simulink model "Computer"  (R2023a)
(part 2 of 6)

  Data_RAM (0x000 .. 0xFFF)/6(b6) -> Word_Enable35/7(b02)
  Data_RAM (0x000 .. 0xFFF)/1(b1) -> Word_Enable35/2(b07)
  Data_RAM (0x000 .. 0xFFF)/8(b8) -> Word_Enable35/9(b00)
  Data_RAM (0x000 .. 0xFFF)/3(b3) -> Word_Enable35/4(b05)
  Data_RAM (0x000 .. 0xFFF)/2(b2) -> Word_Enable35/3(b06)
  Data_ROM (0x000 .. 0xFFF)/2(b2) -> Word_Enable30/3(b06)
  Data_ROM (0x000 .. 0xFFF)/7(b7) -> Word_Enable30/8(b01)
  Data_ROM (0x000 .. 0xFFF)/6(b6) -> Word_Enable30/7(b02)
  Data_ROM (0x000 .. 0xFFF)/4(b4) -> Word_Enable30/5(b04)
  Data_ROM (0x000 .. 0xFFF)/1(b1) -> Word_Enable30/2(b07)
  Data_ROM (0x000 .. 0xFFF)/5(b5) -> Word_Enable30/6(b03)
  Data_ROM (0x000 .. 0xFFF)/3(b3) -> Word_Enable30/4(b05)
  Data_ROM (0x000 .. 0xFFF)/8(b8) -> Word_Enable30/9(b00)
  Word_Enable35/1("b07 ") -> Delay_8b/1
  Word_Enable35/2("b06 ") -> Delay_8b/2
  Word_Enable35/3("b05 ") -> Delay_8b/3
  Word_Enable35/4("b04 ") -> Delay_8b/4
  Word_Enable35/5("b03 ") -> Delay_8b/5
  Word_Enable35/6("b02 ") -> Delay_8b/6
  Word_Enable35/7("b01 ") -> Delay_8b/7
  Word_Enable35/8("b00 ") -> Delay_8b/8
  Merge2_8b_Simulated1/1 -> Merge2_8b_Simulated2/9
  Merge2_8b_Simulated1/2 -> Merge2_8b_Simulated2/10
  Merge2_8b_Simulated1/3 -> Merge2_8b_Simulated2/11
  Merge2_8b_Simulated1/4 -> Merge2_8b_Simulated2/12
  Merge2_8b_Simulated1/5 -> Merge2_8b_Simulated2/13
  Merge2_8b_Simulated1/6 -> Merge2_8b_Simulated2/14
  Merge2_8b_Simulated1/7 -> Merge2_8b_Simulated2/15
  Merge2_8b_Simulated1/8 -> Merge2_8b_Simulated2/16
  Align28/4 -> Video_RAM (0x000 .. 0x3FF)/69(Data_b04)
  Align28/3 -> Video_RAM (0x000 .. 0x3FF)/68(Data_b05)
  Align28/7 -> Video_RAM (0x000 .. 0x3FF)/72(Data_b01)
  Align28/6 -> Video_RAM (0x000 .. 0x3FF)/71(Data_b02)
  Align28/1 -> Video_RAM (0x000 .. 0x3FF)/66(Data_b07)
  Align28/2 -> Video_RAM (0x000 .. 0x3FF)/67(Data_b06)
  Align28/8 -> Video_RAM (0x000 .. 0x3FF)/73(Data_b00)
  Align28/5 -> Video_RAM (0x000 .. 0x3FF)/70(Data_b03)
  Align29/8 -> Align28/8
  Align29/7 -> Align28/7
  Align29/6 -> Align28/6
  Align29/5 -> Align28/5
  Align29/4 -> Align28/4
  Align29/3 -> Align28/3
  Align29/2 -> Align28/2
  Align29/1 -> Align28/1
  <0x2000..0x23FF>/1(Sel(1b)) -> Logical Operator26/2, Word_Enable27/1(Sel(1b))
  Align31/1 -> <0x2000..0x23FF>/1(b15)
  Align31/2 -> <0x2000..0x23FF>/2(b14)
  Align31/3 -> <0x2000..0x23FF>/3(b13)
  Align31/4 -> <0x2000..0x23FF>/4(b12)
  Align31/5 -> <0x2000..0x23FF>/5(b11)
  Align31/6 -> <0x2000..0x23FF>/6(b10), Dec_32_Enbl14/2
  Align31/7 -> Dec_32_Enbl14/3, <0x2000..0x23FF>/7(b09)
  Align31/8 -> <0x2000..0x23FF>/8(b08), Dec_32_Enbl14/4
  Align31/9 -> <0x2000..0x23FF>/9(b07), Dec_32_Enbl14/5
  Align31/10 -> Dec_32_Enbl14/6, <0x2000..0x23FF>/10(b06)
  Align31/11 -> <0x2000..0x23FF>/11(b05)
  Align31/12 -> <0x2000..0x23FF>/12(b04), Align32/5
  Align31/13 -> <0x2000..0x23FF>/13(b03), Align32/4
  Align31/14 -> <0x2000..0x23FF>/14(b02), Align32/3
  Align31/15 -> <0x2000..0x23FF>/15(b01), Align32/2
  Align31/16 -> <0x2000..0x23FF>/16(b00), Align32/1
  Alignment15/1 -> Logical Operator26/1  "Write"
  CLK5/1 -> Video_RAM (0x000 .. 0x3FF)/65(CLK)  "CLK"
  Delay_8b/1 -> Merge2_8b_Simulated1/1
  Delay_8b/2 -> Merge2_8b_Simulated1/2
  Delay_8b/3 -> Merge2_8b_Simulated1/3
  Delay_8b/4 -> Merge2_8b_Simulated1/4
  Delay_8b/5 -> Merge2_8b_Simulated1/5
  Delay_8b/6 -> Merge2_8b_Simulated1/6
  Delay_8b/7 -> Merge2_8b_Simulated1/7
  Delay_8b/8 -> Merge2_8b_Simulated1/8
  Delay_8b1/2 -> Merge2_8b_Simulated2/2
  Delay_8b1/8 -> Merge2_8b_Simulated2/8
  Word_Enable27/7("b01 ") -> Delay_8b1/7
  Word_Enable27/5("b03 ") -> Delay_8b1/5
  Delay_8b1/4 -> Merge2_8b_Simulated2/4
  Delay_8b1/5 -> Merge2_8b_Simulated2/5
  Word_Enable27/1("b07 ") -> Delay_8b1/1
  Word_Enable27/4("b04 ") -> Delay_8b1/4
  Word_Enable27/8("b00 ") -> Delay_8b1/8
  Delay_8b1/3 -> Merge2_8b_Simulated2/3
  Delay_8b1/7 -> Merge2_8b_Simulated2/7
  Delay_8b1/1 -> Merge2_8b_Simulated2/1
  Delay_8b1/6 -> Merge2_8b_Simulated2/6
  Word_Enable27/3("b05 ") -> Delay_8b1/3
  Word_Enable27/6("b02 ") -> Delay_8b1/6
  Word_Enable27/2("b06 ") -> Delay_8b1/2
  Merge2_8b_Simulated2/1 -> Merge2_8b_Simulated9/9
  Merge2_8b_Simulated2/2 -> Merge2_8b_Simulated9/10
  Merge2_8b_Simulated2/3 -> Merge2_8b_Simulated9/11
  Merge2_8b_Simulated2/4 -> Merge2_8b_Simulated9/12
  Merge2_8b_Simulated2/5 -> Merge2_8b_Simulated9/13
  Merge2_8b_Simulated2/6 -> Merge2_8b_Simulated9/14
  Merge2_8b_Simulated2/7 -> Merge2_8b_Simulated9/15
  Merge2_8b_Simulated2/8 -> Merge2_8b_Simulated9/16
  Constant95/1 -> Dec_32_Enbl15/1
  Constant96/1 -> Dec_32_Enbl14/1
  Alignment23/1 -> Alignment15/1
  Word_Enable28/7("b01 ") -> Mux1/7, Merge2_8b_Simulated3/15
  Word_Enable28/2("b06 ") -> Mux1/2, Merge2_8b_Simulated3/10
  Word_Enable28/1("b07 ") -> Mux1/1, Merge2_8b_Simulated3/9
  Word_Enable28/6("b02 ") -> Mux1/6, Merge2_8b_Simulated3/14
  Word_Enable28/4("b04 ") -> Mux1/4, Merge2_8b_Simulated3/12
  Word_Enable28/8("b00 ") -> Mux1/8, Merge2_8b_Simulated3/16
  Word_Enable28/5("b03 ") -> Mux1/5, Merge2_8b_Simulated3/13
  Word_Enable28/3("b05 ") -> Mux1/3, Merge2_8b_Simulated3/11
  Mux1/1 -> Bit to Integer Converter5/1
  Align20/1 -> Align33/1, <0xFFFE..0xFFFE>/1(b15)
  Align20/2 -> Align33/2, <0xFFFE..0xFFFE>/2(b14)
  Align20/3 -> Align33/3, <0xFFFE..0xFFFE>/3(b13)
  Align20/4 -> Align33/4, <0xFFFE..0xFFFE>/4(b12)
  Align20/5 -> Align33/5, <0xFFFE..0xFFFE>/5(b11)
  Align20/6 -> Align33/6, <0xFFFE..0xFFFE>/6(b10)
  Align20/7 -> Align33/7, <0xFFFE..0xFFFE>/7(b09)
  Align20/8 -> Align33/8, <0xFFFE..0xFFFE>/8(b08)
  Align20/9 -> Align33/9, <0xFFFE..0xFFFE>/9(b07)
  Align20/10 -> Align33/10, <0xFFFE..0xFFFE>/10(b06)
  Align20/11 -> Align33/11, <0xFFFE..0xFFFE>/11(b05)
  Align20/12 -> Align33/12, <0xFFFE..0xFFFE>/12(b04)
  Align20/13 -> Align33/13, <0xFFFE..0xFFFE>/13(b03)
  Align20/14 -> Align33/14, <0xFFFE..0xFFFE>/14(b02)
  Align20/15 -> Align33/15, <0xFFFE..0xFFFE>/15(b01)
  Align20/16 -> Align33/16, <0xFFFE..0xFFFE>/16(b00)
  Align34/4 -> Align35/4
  Align34/7 -> Align35/7
  Align34/1 -> Align35/1
  Align34/5 -> Align35/5
  Align34/3 -> Align35/3
  Align34/6 -> Align35/6
  Align34/2 -> Align35/2
  Align34/8 -> Align35/8
  Align35/8 -> Align37/8, Align40/8
  Align35/7 -> Align37/7, Align40/7
  Align35/6 -> Align37/6, Align40/6
  Align35/5 -> Align37/5, Align40/5
  Align35/4 -> Align37/4, Align40/4
  Align35/3 -> Align37/3, Align40/3
  Align35/2 -> Align37/2, Align40/2
  Align35/1 -> Align37/1, Align40/1
  Align37/1 -> Bus Creator2/1
  Align37/2 -> Bus Creator2/2
  Align37/3 -> Bus Creator2/3
  Align37/4 -> Bus Creator2/4
  Align37/5 -> Bus Creator2/5
  Align37/6 -> Bus Creator2/6
  Align37/7 -> Bus Creator2/7
  Align37/8 -> Bus Creator2/8
  Bus Creator2/1 -> Alignment7/1
  Bus Selector6/1 -> Merge2_8b_Simulated3/1  "<b00>"
  Bus Selector6/2 -> Merge2_8b_Simulated3/2  "<b01>"
  Bus Selector6/3 -> Merge2_8b_Simulated3/3  "<b02>"
  Bus Selector6/4 -> Merge2_8b_Simulated3/4  "<b03>"
  Bus Selector6/5 -> Merge2_8b_Simulated3/5  "<b04>"
  Bus Selector6/6 -> Merge2_8b_Simulated3/6  "<b05>"
  Bus Selector6/7 -> Merge2_8b_Simulated3/7  "<b06>"
  Bus Selector6/8 -> Merge2_8b_Simulated3/8  "<b07>"
  Merge2_8b_Simulated3/4 -> Merge2_8b_Simulated4/12
  Merge2_8b_Simulated3/1 -> Merge2_8b_Simulated4/9
  Merge2_8b_Simulated3/6 -> Merge2_8b_Simulated4/14
  Merge2_8b_Simulated3/2 -> Merge2_8b_Simulated4/10
  Merge2_8b_Simulated3/7 -> Merge2_8b_Simulated4/15
  Merge2_8b_Simulated3/3 -> Merge2_8b_Simulated4/11
  Merge2_8b_Simulated3/8 -> Merge2_8b_Simulated4/16
  Merge2_8b_Simulated3/5 -> Merge2_8b_Simulated4/13
  Word_Enable29/1("b07 ") -> Merge2_8b_Simulated4/1
  Word_Enable29/2("b06 ") -> Merge2_8b_Simulated4/2
  Word_Enable29/3("b05 ") -> Merge2_8b_Simulated4/3
  Word_Enable29/4("b04 ") -> Merge2_8b_Simulated4/4
  Word_Enable29/5("b03 ") -> Merge2_8b_Simulated4/5
  Word_Enable29/6("b02 ") -> Merge2_8b_Simulated4/6
  Word_Enable29/7("b01 ") -> Merge2_8b_Simulated4/7
  Word_Enable29/8("b00 ") -> Merge2_8b_Simulated4/8
  Dec_8_Enbl/1 -> Terminator1/1
  Dec_8_Enbl/2 -> Terminator2/1
  Dec_8_Enbl/3 -> Terminator4/1
  Linear_Feedback_Shift_Register_15bit (random number generator)/1(b15) -> Word_Enable32/2(b07)
  Linear_Feedback_Shift_Register_15bit (random number generator)/2(b14) -> Word_Enable32/3(b06)
  Linear_Feedback_Shift_Register_15bit (random number generator)/3(b13) -> Word_Enable32/4(b05)
  Linear_Feedback_Shift_Register_15bit (random number generator)/4(b12) -> Word_Enable32/5(b04)
  Linear_Feedback_Shift_Register_15bit (random number generator)/5(b11) -> Word_Enable32/6(b03)
  Linear_Feedback_Shift_Register_15bit (random number generator)/6(b10) -> Word_Enable32/7(b02)
  Linear_Feedback_Shift_Register_15bit (random number generator)/7(b09) -> Word_Enable32/8(b01)
  Linear_Feedback_Shift_Register_15bit (random number generator)/8(b08) -> Word_Enable32/9(b00)
  <0xFFFF..0xFFFF>/1(Sel(1b)) -> Word_Enable32/1(Sel(1b))
  Align38/1 -> <0xFFFF..0xFFFF>1/1(b15), <0xFFFF..0xFFFF>/1(b15)
  Align38/2 -> <0xFFFF..0xFFFF>/2(b14), <0xFFFF..0xFFFF>1/2(b14)
  Align38/3 -> <0xFFFF..0xFFFF>1/3(b13), <0xFFFF..0xFFFF>/3(b13)
  Align38/4 -> <0xFFFF..0xFFFF>1/4(b12), <0xFFFF..0xFFFF>/4(b12)
  Align38/5 -> <0xFFFF..0xFFFF>1/5(b11), <0xFFFF..0xFFFF>/5(b11)
  Align38/6 -> <0xFFFF..0xFFFF>1/6(b10), <0xFFFF..0xFFFF>/6(b10)
  Align38/7 -> <0xFFFF..0xFFFF>1/7(b09), <0xFFFF..0xFFFF>/7(b09)
  Align38/8 -> <0xFFFF..0xFFFF>1/8(b08), <0xFFFF..0xFFFF>/8(b08)
  Align38/9 -> <0xFFFF..0xFFFF>1/9(b07), <0xFFFF..0xFFFF>/9(b07)
  Align38/10 -> <0xFFFF..0xFFFF>1/10(b06), <0xFFFF..0xFFFF>/10(b06)
  Align38/11 -> <0xFFFF..0xFFFF>1/11(b05), <0xFFFF..0xFFFF>/11(b05)
  Align38/12 -> <0xFFFF..0xFFFF>1/12(b04), <0xFFFF..0xFFFF>/12(b04)
  Align38/13 -> <0xFFFF..0xFFFF>1/13(b03), <0xFFFF..0xFFFF>/13(b03)
  Align38/14 -> <0xFFFF..0xFFFF>1/14(b02), <0xFFFF..0xFFFF>/14(b02)
  Align38/15 -> <0xFFFF..0xFFFF>1/15(b01), <0xFFFF..0xFFFF>/15(b01)
  Align38/16 -> <0xFFFF..0xFFFF>1/16(b00), <0xFFFF..0xFFFF>/16(b00)
  Linear_Feedback_Shift_Register_15bit (random number generator)/9(b07) -> Word_Enable33/2(b07)
  Linear_Feedback_Shift_Register_15bit (random number generator)/13(b03) -> Word_Enable33/6(b03)
  Linear_Feedback_Shift_Register_15bit (random number generator)/11(b05) -> Word_Enable33/4(b05)
  Linear_Feedback_Shift_Register_15bit (random number generator)/12(b04) -> Word_Enable33/5(b04)
  Linear_Feedback_Shift_Register_15bit (random number generator)/15(b01) -> Word_Enable33/8(b01)
  Linear_Feedback_Shift_Register_15bit (random number generator)/10(b06) -> Word_Enable33/3(b06)
  Linear_Feedback_Shift_Register_15bit (random number generator)/16(b00) -> Word_Enable33/9(b00)
  Linear_Feedback_Shift_Register_15bit (random number generator)/14(b02) -> Word_Enable33/7(b02)
  <0xFFFF..0xFFFF>1/1(Sel(1b)) -> Word_Enable33/1(Sel(1b))
  Word_Enable32/8("b00 ") -> Merge2_8b_Simulated5/8
  Word_Enable32/3("b05 ") -> Merge2_8b_Simulated5/3
  Word_Enable32/6("b02 ") -> Merge2_8b_Simulated5/6
  Word_Enable32/1("b07 ") -> Merge2_8b_Simulated5/1
  Word_Enable32/2("b06 ") -> Merge2_8b_Simulated5/2
  Word_Enable32/7("b01 ") -> Merge2_8b_Simulated5/7
  Word_Enable32/4("b04 ") -> Merge2_8b_Simulated5/4
  Word_Enable32/5("b03 ") -> Merge2_8b_Simulated5/5
  Word_Enable33/8("b00 ") -> Merge2_8b_Simulated6/8
  Word_Enable33/3("b05 ") -> Merge2_8b_Simulated6/3
  Word_Enable33/6("b02 ") -> Merge2_8b_Simulated6/6
  Word_Enable33/1("b07 ") -> Merge2_8b_Simulated6/1
  Word_Enable33/2("b06 ") -> Merge2_8b_Simulated6/2
  Word_Enable33/7("b01 ") -> Merge2_8b_Simulated6/7
  Word_Enable33/4("b04 ") -> Merge2_8b_Simulated6/4
  Word_Enable33/5("b03 ") -> Merge2_8b_Simulated6/5
  Merge2_8b_Simulated6/1 -> Merge2_8b_Simulated5/9
  Merge2_8b_Simulated6/2 -> Merge2_8b_Simulated5/10
  Merge2_8b_Simulated6/3 -> Merge2_8b_Simulated5/11
  Merge2_8b_Simulated6/4 -> Merge2_8b_Simulated5/12
  Merge2_8b_Simulated6/5 -> Merge2_8b_Simulated5/13
  Merge2_8b_Simulated6/6 -> Merge2_8b_Simulated5/14
  Merge2_8b_Simulated6/7 -> Merge2_8b_Simulated5/15
  Merge2_8b_Simulated6/8 -> Merge2_8b_Simulated5/16
  Merge2_8b_Simulated5/3 -> Merge2_8b_Simulated7/11
  Merge2_8b_Simulated5/4 -> Merge2_8b_Simulated7/12
  Merge2_8b_Simulated5/8 -> Merge2_8b_Simulated7/16
  Merge2_8b_Simulated5/6 -> Merge2_8b_Simulated7/14
  Merge2_8b_Simulated5/5 -> Merge2_8b_Simulated7/13
  Merge2_8b_Simulated5/1 -> Merge2_8b_Simulated7/9
  Merge2_8b_Simulated5/7 -> Merge2_8b_Simulated7/15
  Merge2_8b_Simulated5/2 -> Merge2_8b_Simulated7/10
  Align39/8 -> Bus Creator10/8
  Align39/7 -> Bus Creator10/7
  Align39/6 -> Bus Creator10/6
  Align39/5 -> Bus Creator10/5
  Align39/2 -> Bus Creator10/2
  Align40/2 -> Align39/2
  Align40/3 -> Align39/3
  Align39/3 -> Bus Creator10/3
  Align40/4 -> Align39/4
  Align40/1 -> Align39/1
  Align40/5 -> Align39/5
  Align40/8 -> Align39/8
  Align40/6 -> Align39/6
  Align40/7 -> Align39/7
  Align39/4 -> Bus Creator10/4
  Align39/1 -> Bus Creator10/1
  Bus Creator10/1 -> Bus Selector15/1, Word_Mux_1/3, StartVal/3, StopVal/3  "CLK(Baudrate)"
  CLK6/1 -> Run/3, Mode/3, StartVal/4, StopVal/4, Counter_Control/7, Counter_16bit/4  "CLK"
  CLK7/1 -> Linear_Feedback_Shift_Register_15bit (random number generator)/1(CLK)  "CLK"
  Bus Selector16/6 -> Word_Enable34/7(b02)  "<b10>"
  Bus Selector16/7 -> Word_Enable34/8(b01)  "<b09>"
  Bus Selector16/8 -> Word_Enable34/9(b00)  "<b08>"
  Bus Selector16/4 -> Word_Enable34/5(b04)  "<b12>"
  Bus Selector16/1 -> Word_Enable34/2(b07)  "<b15>"
  Bus Selector16/3 -> Word_Enable34/4(b05)  "<b13>"
  Bus Selector16/5 -> Word_Enable34/6(b03)  "<b11>"
  Bus Selector16/2 -> Word_Enable34/3(b06)  "<b14>"
  Bus Selector25/1 -> Word_Enable29/2(b07)  "<b07>"
  Bus Selector25/2 -> Word_Enable29/3(b06)  "<b06>"
  Bus Selector25/8 -> Word_Enable29/9(b00)  "<b00>"
  Bus Selector25/7 -> Word_Enable29/8(b01)  "<b01>"
  Bus Selector25/6 -> Word_Enable29/7(b02)  "<b02>"
  Bus Selector25/5 -> Word_Enable29/6(b03)  "<b03>"
  Bus Selector25/4 -> Word_Enable29/5(b04)  "<b04>"
  Bus Selector25/3 -> Word_Enable29/4(b05)  "<b05>"
  Align42/8 -> <0xFFF8..0xFFFD>/8(b08), <0xFFF8..0xFFFD>1/8(b08)
  Align42/11 -> <0xFFF8..0xFFFD>/11(b05), <0xFFF8..0xFFFD>1/11(b05)
  Align42/15 -> <0xFFF8..0xFFFD>/15(b01), <0xFFF8..0xFFFD>1/15(b01), Dec_8_Enbl/3
  Align42/3 -> <0xFFF8..0xFFFD>/3(b13), <0xFFF8..0xFFFD>1/3(b13)
  Align42/16 -> <0xFFF8..0xFFFD>/16(b00), <0xFFF8..0xFFFD>1/16(b00), Dec_8_Enbl/4
  Align42/13 -> <0xFFF8..0xFFFD>/13(b03), <0xFFF8..0xFFFD>1/13(b03)
  Align42/12 -> <0xFFF8..0xFFFD>1/12(b04), <0xFFF8..0xFFFD>/12(b04)
  Align42/9 -> <0xFFF8..0xFFFD>/9(b07), <0xFFF8..0xFFFD>1/9(b07)
  Align42/1 -> <0xFFF8..0xFFFD>1/1(b15), <0xFFF8..0xFFFD>/1(b15)
  Align42/14 -> <0xFFF8..0xFFFD>/14(b02), Dec_8_Enbl/2, <0xFFF8..0xFFFD>1/14(b02)
  Align42/4 -> <0xFFF8..0xFFFD>1/4(b12), <0xFFF8..0xFFFD>/4(b12)
  Align42/2 -> <0xFFF8..0xFFFD>1/2(b14), <0xFFF8..0xFFFD>/2(b14)
  Align42/7 -> <0xFFF8..0xFFFD>/7(b09), <0xFFF8..0xFFFD>1/7(b09)
  Align42/6 -> <0xFFF8..0xFFFD>1/6(b10), <0xFFF8..0xFFFD>/6(b10)
  Align42/10 -> <0xFFF8..0xFFFD>/10(b06), <0xFFF8..0xFFFD>1/10(b06)
  Align42/5 -> <0xFFF8..0xFFFD>1/5(b11), <0xFFF8..0xFFFD>/5(b11)
  <0xFFF8..0xFFFD>/1(Sel(1b)) -> Word_Enable34/1(Sel(1b))
  Merge2_8b_Simulated4/1 -> Merge2_8b_Simulated8/9
  Merge2_8b_Simulated4/2 -> Merge2_8b_Simulated8/10
  Merge2_8b_Simulated4/3 -> Merge2_8b_Simulated8/11
  Merge2_8b_Simulated4/4 -> Merge2_8b_Simulated8/12
  Merge2_8b_Simulated4/5 -> Merge2_8b_Simulated8/13
  Merge2_8b_Simulated4/6 -> Merge2_8b_Simulated8/14
  Merge2_8b_Simulated4/7 -> Merge2_8b_Simulated8/15
  Merge2_8b_Simulated4/8 -> Merge2_8b_Simulated8/16
  Word_Enable34/1("b07 ") -> Merge2_8b_Simulated8/1
  Word_Enable34/2("b06 ") -> Merge2_8b_Simulated8/2
  Word_Enable34/3("b05 ") -> Merge2_8b_Simulated8/3
  Word_Enable34/4("b04 ") -> Merge2_8b_Simulated8/4
  Word_Enable34/5("b03 ") -> Merge2_8b_Simulated8/5
  Word_Enable34/6("b02 ") -> Merge2_8b_Simulated8/6
  Word_Enable34/7("b01 ") -> Merge2_8b_Simulated8/7
  Word_Enable34/8("b00 ") -> Merge2_8b_Simulated8/8
  Merge2_8b_Simulated8/1 -> Merge2_8b_Simulated6/9
  Merge2_8b_Simulated8/2 -> Merge2_8b_Simulated6/10
  Merge2_8b_Simulated8/3 -> Merge2_8b_Simulated6/11
  Merge2_8b_Simulated8/4 -> Merge2_8b_Simulated6/12
  Merge2_8b_Simulated8/5 -> Merge2_8b_Simulated6/13
  Merge2_8b_Simulated8/6 -> Merge2_8b_Simulated6/14
  Merge2_8b_Simulated8/7 -> Merge2_8b_Simulated6/15
  Merge2_8b_Simulated8/8 -> Merge2_8b_Simulated6/16
  Align22/16 -> Align38/16
  Align22/1 -> Align38/1
  Align22/3 -> Align38/3
  Align22/2 -> Align38/2
  Align22/4 -> Align38/4
  Align22/5 -> Align38/5
  Align22/6 -> Align38/6
  Align22/7 -> Align38/7
  Align22/15 -> Align38/15
  Align22/14 -> Align38/14
  Align22/13 -> Align38/13
  Align22/12 -> Align38/12
  Align22/11 -> Align38/11
  Align22/10 -> Align38/10
  Align22/9 -> Align38/9
  Align22/8 -> Align38/8
  Alignment24/1 -> Logical Operator18/6, Mux_4/2
  Alignment25/1 -> Program_Counter/4
  Alignment26/1 -> Mux_4/6
  Program_Counter/1 -> Bus Selector11/1, Bit to Integer Converter15/1  "ProgramCounter"
  Align46/2 -> Align48/2
  Align46/3 -> Align48/1
  Alignment30/1 -> Logical Operator29/2
  Word_Enable36/1("b07 ") -> Merge2_8b_Simulated9/1
  Word_Enable36/2("b06 ") -> Merge2_8b_Simulated9/2
  Word_Enable36/3("b05 ") -> Merge2_8b_Simulated9/3
  Word_Enable36/4("b04 ") -> Merge2_8b_Simulated9/4
  Word_Enable36/5("b03 ") -> Merge2_8b_Simulated9/5
  Word_Enable36/6("b02 ") -> Merge2_8b_Simulated9/6
  Word_Enable36/7("b01 ") -> Merge2_8b_Simulated9/7
  Word_Enable36/8("b00 ") -> Merge2_8b_Simulated9/8
  Merge2_8b_Simulated9/2 -> Merge2_8b_Simulated7/2
  Merge2_8b_Simulated9/6 -> Merge2_8b_Simulated7/6
  Merge2_8b_Simulated9/7 -> Merge2_8b_Simulated7/7
  Merge2_8b_Simulated9/4 -> Merge2_8b_Simulated7/4
  Merge2_8b_Simulated9/5 -> Merge2_8b_Simulated7/5
  Merge2_8b_Simulated9/3 -> Merge2_8b_Simulated7/3
  Merge2_8b_Simulated9/8 -> Merge2_8b_Simulated7/8
  Merge2_8b_Simulated9/1 -> Merge2_8b_Simulated7/1
  Align54/1 -> Align55/3
  Align54/2 -> Align55/2
  Align54/3 -> Align55/1, Word_00/4, Word_01/4, Word_02/4, Word_03/4, Word_04/4, Word_05/4, Word_06/4, Word_07/4, Word_08/4, Word_09/4, Word_10/4, Word_11/4, Word_12/4, Word_13/4, Word_14/4, Word_15/4, Status_Register/1(CLK), Segment_Register/1(Clk), General_Purpose_Register_0/4, General_Purpose_Register_1/4, General_Purpose_Register_2/4, General_Purpose_Register_3/4, General_Purpose_Register_4/4, General_Purpose_Register_5/4, General_Purpose_Register_6/4, General_Purpose_Register_7/4
  Align46/1 -> Align48/3
  Align48/2 -> Align49/2
  Align48/1 -> Align49/3
  Align51/1 -> Alignment23/1, Alignment1/1
  Bus Selector3/1 -> Align46/1  "<RET>"
  Alignment36/1 -> CLK1/1
  Alignment34/1 -> CLK7/1, CLK6/1, CLK3/1
  Alignment35/1 -> CLK2/1, CLK/1
  Align19/2 -> Align10/2, Align17/2
  Align19/12 -> Align10/12, Align17/12
  Align19/10 -> Align10/10, Align17/10
  Align19/1 -> Align10/1, Align17/1
  Align19/15 -> Align10/15, Align17/15
  Align19/14 -> Align10/14, Align17/14
  Align19/3 -> Align10/3, Align17/3
  Align19/16 -> Align10/16, Align17/16
  Align19/6 -> Align10/6, Align17/6
  Align19/8 -> Align10/8, Align17/8
  Align19/5 -> Align10/5, Align17/5
  Align19/7 -> Align10/7, Align17/7
  Align19/9 -> Align10/9, Align17/9
  Align19/4 -> Align10/4, Align17/4
  Align19/13 -> Align10/13, Align17/13
  Align19/11 -> Align10/11, Align17/11
  Bus Selector26/16 -> Align44/1  "<b00>"
  Bus Selector26/15 -> Align44/2  "<b01>"
  Bus Selector26/14 -> Align44/3  "<b02>"
  Bus Selector26/13 -> Align44/4  "<b03>"
  Bus Selector26/12 -> Align44/5  "<b04>"
  Bus Selector26/11 -> Align44/6  "<b05>"
  Bus Selector26/10 -> Align44/7  "<b06>"
  Bus Selector26/9 -> Align44/8  "<b07>"
  Bus Selector26/8 -> Align44/9  "<b08>"
  Bus Selector26/7 -> Align44/10  "<b09>"
  Bus Selector26/6 -> Align44/11  "<b10>"
  Bus Selector26/5 -> Align44/12  "<b11>"
  Bus Selector26/4 -> Align44/13  "<b12>"
  Bus Selector26/3 -> Align44/14  "<b13>"
  Bus Selector26/2 -> Align44/15  "<b14>"
  Bus Selector26/1 -> Align44/16  "<b15>"
  Align44/16 -> Align5/1
  Align44/15 -> Align5/2
  Align44/14 -> Align5/3
  Align44/13 -> Align5/4
  Align44/12 -> Align5/5
  Align44/11 -> Align5/6
  Align44/10 -> Align5/7
  Align44/9 -> Align5/8
  Align44/8 -> Align5/9
  Align44/7 -> Align5/10
  Align44/6 -> Align5/11
  Align44/5 -> Align5/12
  Align44/4 -> Align5/13
  Align44/3 -> Align5/14
  Align44/2 -> Align5/15
  Align44/1 -> Align5/16
  Align5/1 -> Align45/1, Align19/1
  Align5/2 -> Align45/2, Align19/2
  Align5/3 -> Align45/3, Align19/3
  Align5/4 -> Align45/4, Align19/4
  Align5/5 -> Align45/5, Align19/5
  Align5/6 -> Align45/6, Align19/6
  Align5/7 -> Align45/7, Align19/7
  Align5/8 -> Align45/8, Align19/8
  Align5/9 -> Align45/9, Align19/9
  Align5/10 -> Align45/10, Align19/10
  Align5/11 -> Align45/11, Align19/11
  Align5/12 -> Align45/12, Align19/12
  Align5/13 -> Align45/13, Align19/13
  Align5/14 -> Align45/14, Align19/14
  Align5/15 -> Align45/15, Align19/15
  Align5/16 -> Align19/16, Align45/16
  Align17/10 -> Align18/10, Align1/10
  Align17/7 -> Align18/7, Align1/7
  Align17/6 -> Align18/6, Align1/6
  Align17/5 -> Align18/5, Align1/5
  Align17/8 -> Align18/8, Align1/8
  Align17/4 -> Align18/4, Align1/4
  Align17/12 -> Align18/12, Align1/12
  Align17/16 -> Align18/16, Align1/16
  Align17/15 -> Align18/15, Align1/15
  Align17/14 -> Align18/14, Align1/14
  Align17/3 -> Align18/3, Align1/3
  Align17/2 -> Align18/2, Align1/2
  Align17/1 -> Align18/1, Align1/1
  Align17/9 -> Align18/9, Align1/9
  Align17/13 -> Align18/13, Align1/13
  Align17/11 -> Align18/11, Align1/11
  Align1/12 -> Align31/12, Align8/12
  Align1/13 -> Align31/13, Align8/13
  Align1/9 -> Align31/9, Align8/9
  Align1/11 -> Align31/11, Align8/11
  Align1/2 -> Align31/2, Align8/2
  Align1/7 -> Align31/7, Align8/7
  Align1/14 -> Align31/14, Align8/14
  Align1/16 -> Align31/16, Align8/16
  Align1/4 -> Align31/4, Align8/4
  Align1/5 -> Align31/5, Align8/5
  Align1/10 -> Align31/10, Align8/10
  Align1/6 -> Align31/6, Align8/6
  Align1/8 -> Align31/8, Align8/8
  Align1/15 -> Align8/15, Align31/15
  Align1/1 -> Align31/1, Align8/1
  Align1/3 -> Align31/3, Align8/3
  Align8/16 -> <0xFFF7..0xFFF7>/16(b00)
  Align8/15 -> <0xFFF7..0xFFF7>/15(b01)
  Align8/14 -> <0xFFF7..0xFFF7>/14(b02)
  Align8/13 -> <0xFFF7..0xFFF7>/13(b03)
  Align8/12 -> <0xFFF7..0xFFF7>/12(b04)
  Align8/11 -> <0xFFF7..0xFFF7>/11(b05)
  Align8/10 -> <0xFFF7..0xFFF7>/10(b06)
  Align8/9 -> <0xFFF7..0xFFF7>/9(b07)
  Align8/8 -> <0xFFF7..0xFFF7>/8(b08)
  Align8/7 -> <0xFFF7..0xFFF7>/7(b09)
  Align8/6 -> <0xFFF7..0xFFF7>/6(b10)
  Align8/5 -> <0xFFF7..0xFFF7>/5(b11)
  Align8/4 -> <0xFFF7..0xFFF7>/4(b12)
  Align8/3 -> <0xFFF7..0xFFF7>/3(b13)
  Align8/2 -> <0xFFF7..0xFFF7>/2(b14)
  Align8/1 -> <0xFFF7..0xFFF7>/1(b15)
  Bus Selector4/8 -> Align21/1  "<b00>"
  Bus Selector4/7 -> Align21/2  "<b01>"
  Bus Selector4/6 -> Align21/3  "<b02>"
  Bus Selector4/5 -> Align21/4  "<b03>"
  Bus Selector4/4 -> Align21/5  "<b04>"
  Bus Selector4/3 -> Align21/6  "<b05>"
  Bus Selector4/2 -> Align21/7  "<b06>"
  Bus Selector4/1 -> Align21/8  "<b07>"
  Align21/8 -> Align24/1
  Align21/7 -> Align24/2
  Align21/6 -> Align24/3
  Align21/5 -> Align24/4
  Align21/4 -> Align24/5
  Align21/3 -> Align24/6
  Align21/2 -> Align24/7
  Align21/1 -> Align24/8
  Align30/4 -> Align29/4, Align27/4
  Align43/2 -> Align25/2, Align30/2
  Align30/8 -> Align29/8, Align27/8
  Align27/4 -> Align36/4
  Align27/5 -> Align36/5
  Align27/2 -> Align36/2
  Align43/3 -> Align25/3, Align30/3
  Align27/8 -> Align36/8
  Align30/6 -> Align29/6, Align27/6
  Align43/4 -> Align25/4, Align30/4
  Align43/7 -> Align25/7, Align30/7
  Align43/5 -> Align25/5, Align30/5
  Align27/3 -> Align36/3
  Align43/8 -> Align25/8, Align30/8
  Align43/1 -> Align25/1, Align30/1
  Align43/6 -> Align25/6, Align30/6
  Align27/6 -> Align36/6
  Align27/1 -> Align36/1
  Align27/7 -> Align36/7
  Align30/3 -> Align29/3, Align27/3
  Align30/5 -> Align29/5, Align27/5
  Align30/7 -> Align29/7, Align27/7
  Align30/2 -> Align29/2, Align27/2
  Align30/1 -> Align29/1, Align27/1
  Align24/1 -> Align34/1, Align43/1
  Align24/2 -> Align34/2, Align43/2
  Align24/3 -> Align34/3, Align43/3
  Align24/4 -> Align34/4, Align43/4
  Align24/5 -> Align34/5, Align43/5
  Align24/6 -> Align34/6, Align43/6
  Align24/7 -> Align34/7, Align43/7
  Align24/8 -> Align34/8, Align43/8
  Align36/6 -> Align41/6
  Align36/1 -> Align41/1
  Align36/3 -> Align41/3
  Align36/2 -> Align41/2
  Align36/4 -> Align41/4
  Align36/8 -> Align41/8
  Align36/7 -> Align41/7
  Align36/5 -> Align41/5
  Align48/3 -> Align49/1
  Align49/1 -> Align50/1
  Align49/2 -> Align50/2
  Align49/3 -> Align50/3
  Align50/1 -> Align51/1
  Align50/2 -> Align51/2
  Align50/3 -> Align51/3
  Align47/1 -> Align54/1
  Align47/2 -> Align54/2
  Align47/3 -> Align54/3
  Align56/1 -> Alignment5/1, CLK5/1, CLK4/1, Alignment34/1, Alignment35/1
  Align56/3 -> Alignment36/1
  Align55/3 -> Align56/1
  Align55/2 -> Align56/2
  Align55/1 -> Align56/3
  Align56/2 -> ?
  Bus Creator11/1 -> Select_Address/6  "Status"
  AuxALU/1 -> Bus Selector18/1
  Bus Creator12/1 -> Word_Mux_4(6)/6  "Status"
  Bus Selector18/1 -> Align58/1  "<b15>"
  Bus Selector18/16 -> Align58/16  "<b00>"
  Bus Selector18/15 -> Align58/15  "<b01>"
  Bus Selector18/14 -> Align58/14  "<b02>"
  Bus Selector18/13 -> Align58/13  "<b03>"
  Bus Selector18/12 -> Align58/12  "<b04>"
  Bus Selector18/11 -> Align58/11  "<b05>"
  Bus Selector18/10 -> Align58/10  "<b06>"
  Bus Selector18/9 -> Align58/9  "<b07>"
  Bus Selector18/8 -> Align58/8  "<b08>"
  Bus Selector18/7 -> Align58/7  "<b09>"
  Bus Selector18/6 -> Align58/6  "<b10>"
  Bus Selector18/5 -> Align58/5  "<b11>"
  Bus Selector18/4 -> Align58/4  "<b12>"
  Bus Selector18/3 -> Align58/3  "<b13>"
  Bus Selector18/2 -> Align58/2  "<b14>"
  Align58/1 -> Bus Creator11/1, Align59/1
  Align58/2 -> Bus Creator11/2, Align59/2
  Align58/3 -> Bus Creator11/3, Align59/3
  Align58/4 -> Bus Creator11/4, Align59/4
  Align58/5 -> Bus Creator11/5, Align59/5
  Align58/6 -> Bus Creator11/6, Align59/6
  Align58/7 -> Bus Creator11/7, Align59/7
  Align58/8 -> Bus Creator11/8, Align59/8
  Align58/9 -> Bus Creator11/9, Align59/9
  Align58/10 -> Bus Creator11/10, Align59/10
  Align58/11 -> Bus Creator11/11, Align59/11
  Align58/12 -> Bus Creator11/12, Align59/12
  Align58/13 -> Bus Creator11/13, Align59/13
  Align58/14 -> Bus Creator11/14, Align59/14
  Align58/15 -> Bus Creator11/15, Align59/15
  Align58/16 -> Bus Creator11/16, Align59/16
  Align59/15 -> Bus Creator12/15
  Align59/14 -> Bus Creator12/14
  Align59/13 -> Bus Creator12/13
  Align59/12 -> Bus Creator12/12
  Align59/11 -> Bus Creator12/11
  Align59/10 -> Bus Creator12/10
  Align59/9 -> Bus Creator12/9
  Align59/8 -> Bus Creator12/8
  Align59/7 -> Bus Creator12/7
  Align59/6 -> Bus Creator12/6
  Align59/5 -> Bus Creator12/5
  Align59/4 -> Bus Creator12/4
  Align59/3 -> Bus Creator12/3
  Align59/2 -> Bus Creator12/2
  Align59/1 -> Bus Creator12/1
  Align63/1 -> Align65/1
  Align63/2 -> Align65/2
  Align63/3 -> Align65/3
  Align63/4 -> Align65/4
  Align63/5 -> Align65/5
  Align63/6 -> Align65/6
  Align63/7 -> Align65/7
  Align63/8 -> Align65/8
  Align63/9 -> Align65/9
  Align63/10 -> Align65/10
  Align63/11 -> Align65/11
  Align63/12 -> Align65/12
  Bus Selector11/1 -> Align64/1, Align69/12  "<b11>"
  Bus Selector11/2 -> Align64/2, Align69/11  "<b10>"
  Bus Selector11/12 -> Align64/12, Align69/1  "<b00>"
  Bus Selector11/11 -> Align64/11, Align69/2  "<b01>"
  Bus Selector11/10 -> Align64/10, Align69/3  "<b02>"
  Bus Selector11/9 -> Align64/9, Align69/4  "<b03>"
  Bus Selector11/8 -> Align64/8, Align69/5  "<b04>"
  Bus Selector11/7 -> Align64/7, Align69/6  "<b05>"
  Bus Selector11/6 -> Align64/6, Align69/7  "<b06>"
  Bus Selector11/5 -> Align64/5, Align69/8  "<b07>"
  Bus Selector11/4 -> Align64/4, Align69/9  "<b08>"
  Bus Selector11/3 -> Align64/3, Align69/10  "<b09>"
  Bus Creator13/1 -> Word_Mux_5/4  "Status"
  Align64/10 -> Bus Creator13/14
  Align64/9 -> Bus Creator13/13
  Align64/8 -> Bus Creator13/12
  Align64/12 -> Bus Creator13/16
  Align64/3 -> Bus Creator13/7
  Align64/7 -> Bus Creator13/11
  Align64/5 -> Bus Creator13/9
  Align64/11 -> Bus Creator13/15
  Align64/6 -> Bus Creator13/10
  Align64/2 -> Bus Creator13/6
  Align64/4 -> Bus Creator13/8
  Align64/1 -> Bus Creator13/5
  Align65/1 -> Align67/1
  Align65/2 -> Align67/2
  Align65/3 -> Align67/3
  Align65/4 -> Align67/4
  Align65/5 -> Align67/5
  Align65/6 -> Align67/6
  Align65/7 -> Align67/7
  Align65/8 -> Align67/8
  Align65/9 -> Align67/9
  Align65/10 -> Align67/10
  Align65/11 -> Align67/11
  Align65/12 -> Align67/12
  Align67/12 -> Align68/12, Align4/12
  Align67/11 -> Align68/11, Align4/11
  Align67/10 -> Align68/10, Align4/10
  Align67/9 -> Align68/9, Align4/9
  Align67/8 -> Align68/8, Align4/8
  Align67/7 -> Align68/7, Align4/7
  Align67/6 -> Align68/6, Align4/6
  Align67/5 -> Align68/5, Align4/5
  Align67/4 -> Align68/4, Align4/4
  Align67/3 -> Align68/3, Align4/3
  Align67/2 -> Align68/2, Align4/2
  Align67/1 -> Align68/1, Align4/1
  Align68/1 -> Bus Creator14/5
  Align68/11 -> Bus Creator14/15
  Align68/2 -> Bus Creator14/6
  Align68/3 -> Bus Creator14/7
  Align68/7 -> Bus Creator14/11
  Align68/5 -> Bus Creator14/9
  Align68/4 -> Bus Creator14/8
  Align68/10 -> Bus Creator14/14
  Align68/8 -> Bus Creator14/12
  Align68/6 -> Bus Creator14/10
  Align68/9 -> Bus Creator14/13
  Align68/12 -> Bus Creator14/16
  Bus Creator14/1 -> Word_Mux_4(6)/8  "Status"
  Align69/1 -> Align85/1
  Align69/2 -> Align85/2
  Align69/3 -> Align85/3
  Align69/4 -> Align85/4
  Align69/5 -> Align85/5
  Align69/6 -> Align85/6
  Align69/7 -> Align85/7
  Align69/8 -> Align85/8
  Align69/9 -> Align85/9
  Align69/10 -> Align85/10
  Align69/11 -> Align85/11
  Align69/12 -> Align85/12
  Bus Creator15/1 -> Word_Mux_3/8  "Immediate"
  Bus Creator16/1 -> Mux_4/7  "Status"
  Bus Creator17/1 -> Word_Mux_5/3  "Status"
  Bus Creator18/1 -> Segment_Register/4(Addr(2B)), Word_Mux_7/8
  Bus Selector27/12 -> Align73/1, Align66/12  "<b00>"
  Bus Selector27/1 -> Align73/12, Align66/1  "<b11>"
  Bus Selector27/2 -> Align73/11, Align66/2  "<b10>"
  Bus Selector27/3 -> Align73/10, Align66/3  "<b09>"
  Bus Selector27/11 -> Align73/2, Align66/11  "<b01>"
  Bus Selector27/10 -> Align73/3, Align66/10  "<b02>"
  Bus Selector27/9 -> Align73/4, Align66/9  "<b03>"
  Bus Selector27/8 -> Align73/5, Align66/8  "<b04>"
  Bus Selector27/7 -> Align73/6, Align66/7  "<b05>"
  Bus Selector27/6 -> Align73/7, Align66/6  "<b06>"
  Bus Selector27/5 -> Align73/8, Align66/5  "<b07>"
  Bus Selector27/4 -> Align73/9, Align66/4  "<b08>"
  Align66/12 -> Bus Creator18/12
  Align66/11 -> Bus Creator18/11
  Align66/10 -> Bus Creator18/10
  Align66/9 -> Bus Creator18/9
  Align66/8 -> Bus Creator18/8
  Align66/7 -> Bus Creator18/7
  Align66/6 -> Bus Creator18/6
  Align66/5 -> Bus Creator18/5
  Align66/4 -> Bus Creator18/4
  Align66/3 -> Bus Creator18/3
  Align66/2 -> Bus Creator18/2
  Align66/1 -> Bus Creator18/1
  Align70/1 -> Bus Creator17/12
  Align70/2 -> Bus Creator17/11
  Align70/3 -> Bus Creator17/10
  Align70/4 -> Bus Creator17/9
  Align70/5 -> Bus Creator17/8
  Align70/6 -> Bus Creator17/7
  Align70/7 -> Bus Creator17/6
  Align70/8 -> Bus Creator17/5
  Align70/9 -> Bus Creator17/4
  Align70/10 -> Bus Creator17/3
  Align70/11 -> Bus Creator17/2
  Align70/12 -> Bus Creator17/1
  Align72/1 -> Align62/1, Bus Creator16/12
  Align72/2 -> Align62/2, Bus Creator16/11
  Align72/3 -> Align62/3, Bus Creator16/10
  Align72/4 -> Align62/4, Bus Creator16/9
  Align72/5 -> Align62/5, Bus Creator16/8
  Align72/6 -> Align62/6, Bus Creator16/7
  Align72/7 -> Align62/7, Bus Creator16/6
  Align72/8 -> Align62/8, Bus Creator16/5
  Align72/9 -> Align62/9, Bus Creator16/4
  Align72/10 -> Align62/10, Bus Creator16/3
  Align72/11 -> Align62/11, Bus Creator16/2
  Align72/12 -> Align62/12, Bus Creator16/1
  Bus Creator19/1 -> Status_Register/3(Status(2B))
  Align74/4 -> Align75/4  "Status"
  Align74/3 -> Align75/3
  Align74/2 -> Align75/2
  Align74/1 -> Align75/1
  Align75/4 -> Align76/1
  Align75/3 -> Align76/2
  Align75/2 -> Align76/3
  Align75/1 -> Align76/4
  Align76/4 -> Align77/4
  Align76/3 -> Align77/3
  Align76/2 -> Align77/2
  Align77/4 -> Bus Creator19/1
  Align77/3 -> Bus Creator19/2
  Align77/2 -> Bus Creator19/3
  Align77/1 -> Bus Creator19/4
  Merge16_Simulated/1 -> Bus Selector28/1  "ALU"
  Bus Creator20/1 -> "Select_Data  "/4  "Status"
  Bus Creator21/1 -> Word_Mux_7/5  "Status"
  Align78/16 -> Align79/1
  Align79/1 -> Align80/1
  Align78/15 -> Align79/2
  Align78/14 -> Align79/3
  Align78/13 -> Align79/4
  Align78/12 -> Align79/5
  Align78/11 -> Align79/6
  Align78/10 -> Align79/7
  Align78/9 -> Align79/8
  Align78/8 -> Align79/9
  Align78/7 -> Align79/10
  Align78/6 -> Align79/11
  Align78/5 -> Align79/12
  Align78/4 -> Align79/13
  Align78/3 -> Align79/14
  Align78/2 -> Align79/15
  Align78/1 -> Align79/16
  Bus Selector28/15 -> Align81/7, Align78/15  "<b01>"
  Bus Selector28/14 -> Align78/14, Align81/6  "<b02>"
  Bus Selector28/13 -> Align78/13, Align81/5  "<b03>"
  Bus Selector28/12 -> Align78/12, Align81/4  "<b04>"
  Bus Selector28/11 -> Align78/11, Align81/3  "<b05>"
  Bus Selector28/10 -> Align78/10, Align81/2  "<b06>"
  Bus Selector28/9 -> Align78/9, Align81/1  "<b07>"
  Bus Selector28/8 -> Align78/8  "<b08>"
  Bus Selector28/7 -> Align78/7  "<b09>"
  Bus Selector28/6 -> Align78/6  "<b10>"
  Bus Selector28/5 -> Align78/5  "<b11>"
  Bus Selector28/4 -> Align78/4  "<b12>"
  Bus Selector28/3 -> Align78/3  "<b13>"
  Bus Selector28/2 -> Align78/2  "<b14>"
  Bus Selector28/1 -> Align78/1  "<b15>"
  Align79/2 -> Align80/2
  Align79/3 -> Align80/3
  Align79/4 -> Align80/4
  Align79/5 -> Align80/5
  Align79/6 -> Align80/6
  Align79/7 -> Align80/7
  Align79/8 -> Align80/8
  Align79/9 -> Align80/9
  Align79/10 -> Align80/10
  Align79/11 -> Align80/11
  Align79/12 -> Align80/12
  Align79/13 -> Align80/13
  Align79/14 -> Align80/14
  Align79/15 -> Align80/15
  Align79/16 -> Align80/16
  Align81/1 -> Bus Creator20/1
  Align81/2 -> Bus Creator20/2
  Align81/3 -> Bus Creator20/3
  Align81/4 -> Bus Creator20/4
  Align81/5 -> Bus Creator20/5
  Align81/6 -> Bus Creator20/6
  Align81/7 -> Bus Creator20/7
  Align81/8 -> Bus Creator20/8
  Bus Selector29/3 -> Align57/3  "<b00>"
  Bus Selector29/2 -> Align57/2  "<b01>"
  Bus Selector29/1 -> Align57/1  "<b02>"
  Bus Selector30/1 -> Align82/1  "<b02>"
  Bus Selector30/2 -> Align82/2  "<b01>"
  Bus Selector30/3 -> Align82/3  "<b00>"
  Align57/3 -> Align83/3
  Align57/2 -> Align83/2
  Align57/1 -> Align83/1
  Align82/3 -> Align84/3
  Align82/2 -> Align84/2
  Align82/1 -> Align84/1
  Align3/12 -> Align70/1
  Align3/11 -> Align70/2
  Align3/10 -> Align70/3
  Align3/9 -> Align70/4
  Align3/8 -> Align70/5
  Align3/7 -> Align70/6
  Align3/6 -> Align70/7
  Align3/5 -> Align70/8
  Align3/4 -> Align70/9
  Align3/3 -> Align70/10
  Align3/2 -> Align70/11
  Align3/1 -> Align70/12
  Align73/5 -> Align72/5, Align3/8
  Align73/6 -> Align72/6, Align3/7
  Align73/10 -> Align72/10, Align3/3
  Align73/12 -> Align72/12, Align3/1
  Align73/11 -> Align72/11, Align3/2
  Align73/9 -> Align72/9, Align3/4
  Align73/2 -> Align72/2, Align3/11
  Align73/4 -> Align72/4, Align3/9
  Align73/3 -> Align72/3, Align3/10
  Align73/8 -> Align72/8, Align3/5
  Align73/7 -> Align72/7, Align3/6
  Align73/1 -> Align72/1, Align3/12
  Align85/1 -> Align63/1
  Align85/2 -> Align63/2
  Align85/3 -> Align63/3
  Align85/4 -> Align63/4
  Align85/5 -> Align63/5
  Align85/6 -> Align63/6
  Align85/7 -> Align63/7
  Align85/8 -> Align63/8
  Align85/9 -> Align63/9
  Align85/10 -> Align63/10
  Align85/11 -> Align63/11
  Align85/12 -> Align63/12
  Bus Selector13/1 -> Bus Creator22/1, Align86/16  "<b15>"
  Bus Selector13/2 -> Bus Creator22/2, Align86/15  "<b14>"
  Bus Selector13/3 -> Bus Creator22/3, Align86/14  "<b13>"
  Bus Selector13/4 -> Bus Creator22/4, Align86/13  "<b12>"
  Bus Selector13/5 -> Bus Creator22/5, Align86/12  "<b11>"
  Bus Selector13/6 -> Bus Creator22/6, Align86/11  "<b10>"
  Bus Selector13/7 -> Bus Creator22/7, Align86/10  "<b09>"
  Bus Selector13/8 -> Bus Creator22/8, Align86/9  "<b08>"
  Bus Selector13/9 -> Bus Creator22/9, Align86/8  "<b07>"
  Bus Selector13/10 -> Bus Creator22/10, Align86/7  "<b06>"
  Bus Selector13/11 -> Bus Creator22/11, Align86/6  "<b05>"
  Bus Selector13/12 -> Bus Creator22/12, Align86/5  "<b04>"
  Bus Selector13/13 -> Bus Creator22/13, Align86/4  "<b03>"
  Bus Selector13/14 -> Bus Creator22/14, Align86/3  "<b02>"
  Bus Selector13/15 -> Bus Creator22/15, Align86/2  "<b01>"
  Bus Selector13/16 -> Bus Creator22/16, Align86/1  "<b00>"
  Align86/1 -> Align88/1, Bus Creator23/16
  Align86/2 -> Align88/2, Bus Creator23/15
  Align86/3 -> Align88/3, Bus Creator23/14
  Align86/4 -> Align88/4, Bus Creator23/13
  Align86/5 -> Align88/5, Bus Creator23/12
  Align86/6 -> Align88/6, Bus Creator23/11
  Align86/7 -> Align88/7, Bus Creator23/10
  Align86/8 -> Align88/8, Bus Creator23/9
  Align86/9 -> Align88/9, Bus Creator23/8
  Align86/10 -> Align88/10, Bus Creator23/7
  Align86/11 -> Align88/11, Bus Creator23/6
  Align86/12 -> Align88/12, Bus Creator23/5
  Align86/13 -> Align88/13, Bus Creator23/4
  Align86/14 -> Align88/14, Bus Creator23/3
  Align86/15 -> Align88/15, Bus Creator23/2
  Align86/16 -> Align88/16, Bus Creator23/1
  Bus Creator24/1 -> Word_Mux_2/7, Word_Mux_3/7  "SrcRegVal"
  Merge8_Simulated1/1 -> Bus Selector1/1  "DestRegVal"
  Bus Selector1/16 -> Align89/1  "<b00>"
  Bus Selector1/15 -> Align89/2  "<b01>"
  Bus Selector1/14 -> Align89/3  "<b02>"
  Bus Selector1/13 -> Align89/4  "<b03>"
  Bus Selector1/12 -> Align89/5  "<b04>"
  Bus Selector1/11 -> Align89/6  "<b05>"
  Bus Selector1/10 -> Align89/7  "<b06>"
  Bus Selector1/9 -> Align89/8  "<b07>"
  Bus Selector1/8 -> Align89/9  "<b08>"
  Bus Selector1/7 -> Align89/10  "<b09>"
  Bus Selector1/6 -> Align89/11  "<b10>"
  Bus Selector1/5 -> Align89/12  "<b11>"
  Bus Selector1/4 -> Align89/13  "<b12>"
  Bus Selector1/3 -> Align89/14  "<b13>"
  Bus Selector1/2 -> Align89/15  "<b14>"
  Bus Selector1/1 -> Align89/16  "<b15>"
  Align89/1 -> Align90/1, Bus Creator26/16
  Align89/2 -> Align90/2, Bus Creator26/15
  Align89/3 -> Align90/3, Bus Creator26/14
  Align89/4 -> Align90/4, Bus Creator26/13
  Align89/5 -> Align90/5, Bus Creator26/12
  Align89/6 -> Align90/6, Bus Creator26/11
  Align89/7 -> Align90/7, Bus Creator26/10
  Align89/8 -> Align90/8, Bus Creator26/9
  Align89/9 -> Align90/9, Bus Creator26/8
  Align89/10 -> Align90/10, Bus Creator26/7
  Align89/11 -> Align90/11, Bus Creator26/6
  Align89/12 -> Align90/12, Bus Creator26/5
  Align89/13 -> Align90/13, Bus Creator26/4
  Align89/14 -> Align90/14, Bus Creator26/3
  Align89/15 -> Align90/15, Bus Creator26/2
  Align89/16 -> Align90/16, Bus Creator26/1
  Merge2_8b_Simulated7/1 -> Align92/8
  Merge2_8b_Simulated7/2 -> Align92/7
  Merge2_8b_Simulated7/3 -> Align92/6
  Merge2_8b_Simulated7/4 -> Align92/5
  Merge2_8b_Simulated7/5 -> Align92/4
  Merge2_8b_Simulated7/6 -> Align92/3
  Merge2_8b_Simulated7/7 -> Align92/2
  Merge2_8b_Simulated7/8 -> Align92/1
  Align92/8 -> Bus Creator27/1, Align95/8
  Align92/7 -> Bus Creator27/2, Align95/7
  Align92/6 -> Bus Creator27/3, Align95/6
  Align92/5 -> Bus Creator27/4, Align95/5
  Align92/4 -> Bus Creator27/5, Align95/4
  Align92/3 -> Bus Creator27/6, Align95/3
  Align92/2 -> Bus Creator27/7, Align95/2
  Align92/1 -> Bus Creator27/8, Align95/1
  Align4/1 -> Align97/12
  Align4/2 -> Align97/11
  Align4/3 -> Align97/10
  Align4/4 -> Align97/9
  Align4/5 -> Align97/8
  Align4/6 -> Align97/7
  Align4/7 -> Align97/6
  Align4/8 -> Align97/5
  Align4/9 -> Align97/4
  Align4/10 -> Align97/3
  Align4/11 -> Align97/2
  Align4/12 -> Align97/1
  Align97/12 -> Align98/12
  Align97/11 -> Align98/11
  Align97/10 -> Align98/10
  Align97/9 -> Align98/9
  Align97/8 -> Align98/8
  Align97/7 -> Align98/7
  Align97/6 -> Align98/6
  Align97/5 -> Align98/5
  Align97/4 -> Align98/4
  Align97/3 -> Align98/3
  Align97/2 -> Align98/2
  Align97/1 -> Align98/1
  Align98/12 -> Align61/1
  Align98/11 -> Align61/2
  Align98/10 -> Align61/3
  Align98/9 -> Align61/4
  Align98/8 -> Align61/5
  Align98/7 -> Align61/6
  Align98/6 -> Align61/7
  Align98/5 -> Align61/8
  Align98/4 -> Align61/9
  Align98/3 -> Align61/10
  Align98/2 -> Align61/11
  Align98/1 -> Align61/12
  Align88/16 -> Bus Creator24/1
  Align88/15 -> Bus Creator24/2
  Align88/14 -> Bus Creator24/3
  Align88/13 -> Bus Creator24/4
  Align88/12 -> Bus Creator24/5
  Align88/11 -> Bus Creator24/6
  Align88/10 -> Bus Creator24/7
  Align88/9 -> Bus Creator24/8
  Align88/8 -> Bus Creator24/9
  Align88/7 -> Bus Creator24/10
  Align88/6 -> Bus Creator24/11
  Align88/5 -> Bus Creator24/12
  Align88/4 -> Bus Creator24/13
  Align88/3 -> Bus Creator24/14
  Align88/2 -> Bus Creator24/15
  Align88/1 -> Bus Creator24/16
  Align90/16 -> Bus Creator25/1
  Align90/15 -> Bus Creator25/2
  Align90/14 -> Bus Creator25/3
  Align90/13 -> Bus Creator25/4
  Align90/12 -> Bus Creator25/5
  Align90/11 -> Bus Creator25/6
  Align90/10 -> Bus Creator25/7
  Align90/9 -> Bus Creator25/8
  Align90/8 -> Bus Creator25/9
  Align90/7 -> Bus Creator25/10
  Align90/6 -> Bus Creator25/11
  Align90/5 -> Bus Creator25/12
  Align90/4 -> Bus Creator25/13
  Align90/3 -> Bus Creator25/14
  Align90/2 -> Bus Creator25/15
  Align90/1 -> Bus Creator25/16
  Align60/1 -> Bus Creator15/1
  Align60/2 -> Bus Creator15/2
  Align60/3 -> Bus Creator15/3
  Align60/4 -> Bus Creator15/4
  Align60/5 -> Bus Creator15/5
  Align60/6 -> Bus Creator15/6
  Align60/7 -> Bus Creator15/7
  Align60/8 -> Bus Creator15/8
  Align60/9 -> Bus Creator15/9
  Align60/10 -> Bus Creator15/10
  Align60/11 -> Bus Creator15/11
  Align60/12 -> Bus Creator15/12
  Align62/12 -> Align60/1
  Align62/11 -> Align60/2
  Align62/10 -> Align60/3
  Align62/9 -> Align60/4
  Align62/8 -> Align60/5
  Align62/7 -> Align60/6
  Align62/6 -> Align60/7
  Align62/5 -> Align60/8
  Align62/4 -> Align60/9
  Align62/3 -> Align60/10
  Align62/2 -> Align60/11
  Align62/1 -> Align60/12
  Align80/16 -> Bus Creator21/1
  Align80/15 -> Bus Creator21/2
  Align80/14 -> Bus Creator21/3
  Align80/13 -> Bus Creator21/4
  Align80/12 -> Bus Creator21/5
  Align80/11 -> Bus Creator21/6
  Align80/10 -> Bus Creator21/7
  Align80/9 -> Bus Creator21/8
  Align80/8 -> Bus Creator21/9
  Align80/7 -> Bus Creator21/10
  Align80/6 -> Bus Creator21/11
  Align80/5 -> Bus Creator21/12
  Align80/4 -> Bus Creator21/13
  Align80/3 -> Bus Creator21/14
  Align80/2 -> Bus Creator21/15
  Align80/1 -> Bus Creator21/16
  Bus Selector17/1 -> Align91/2  "<Equal>"
  Bus Selector17/2 -> Align91/1  "<LessThanSigned>"
  Align91/2 -> Align71/1
  Align91/1 -> Align71/2
  Bus Selector9/1 -> Align87/1  "<b15>"
  Bus Selector9/16 -> Align87/16  "<b00>"
  Bus Selector9/15 -> Align87/15  "<b01>"
  Bus Selector9/14 -> Align87/14  "<b02>"
  Bus Selector9/13 -> Align87/13  "<b03>"
  Bus Selector9/12 -> Align87/12  "<b04>"
  Bus Selector9/11 -> Align87/11  "<b05>"
  Bus Selector9/10 -> Align87/10  "<b06>"
  Bus Selector9/9 -> Align87/9  "<b07>"
  Bus Selector9/8 -> Align87/8  "<b08>"
  Bus Selector9/7 -> Align87/7  "<b09>"
  Bus Selector9/6 -> Align87/6  "<b10>"
  Bus Selector9/5 -> Align87/5  "<b11>"
  Bus Selector9/4 -> Align87/4  "<b12>"
  Bus Selector9/3 -> Align87/3  "<b13>"
  Bus Selector9/2 -> Align87/2  "<b14>"
  Align87/1 -> Align99/16
  Align87/2 -> Align99/15
  Align87/3 -> Align99/14
  Align87/4 -> Align99/13
  Align87/5 -> Align99/12
  Align87/6 -> Align99/11
  Align87/7 -> Align99/10
  Align87/8 -> Align99/9
  Align87/9 -> Align99/8
  Align87/10 -> Align99/7
  Align87/11 -> Align99/6
  Align87/12 -> Align99/5
  Align87/13 -> Align99/4
  Align87/14 -> Align99/3
  Align87/15 -> Align99/2
  Align87/16 -> Align99/1
  Align99/16 -> Align100/16
  Align99/15 -> Align100/15
  Align99/14 -> Align100/14
  Align99/13 -> Align100/13
  Align99/12 -> Align100/12
  Align99/11 -> Align100/11
  Align99/10 -> Align100/10
  Align99/9 -> Align100/9
  Align99/8 -> Align100/8
  Align99/7 -> Align100/7
  Align99/6 -> Align100/6
  Align99/5 -> Align100/5
  Align99/4 -> Align100/4
  Align99/3 -> Align100/3
  Align99/2 -> Align100/2
  Align99/1 -> Align100/1
  Align100/16 -> Align101/16, Bus Creator1/1
  Align100/15 -> Bus Creator1/2, Align101/15
  Align100/14 -> Bus Creator1/3, Align101/14
  Align100/13 -> Bus Creator1/4, Align101/13
  Align100/12 -> Bus Creator1/5, Align101/12
  Align100/11 -> Bus Creator1/6, Align101/11
  Align100/10 -> Bus Creator1/7, Align101/10
  Align100/9 -> Bus Creator1/8, Align101/9
  Align100/8 -> Bus Creator1/9, Align101/8
  Align100/7 -> Bus Creator1/10, Align101/7
  Align100/6 -> Bus Creator1/11, Align101/6
  Align100/5 -> Bus Creator1/12, Align101/5
  Align100/4 -> Bus Creator1/13, Align101/4
  Align100/3 -> Bus Creator1/14, Align101/3
  Align100/2 -> Bus Creator1/15, Align101/2
  Align100/1 -> Bus Creator1/16, Align101/1
  Bus Creator1/1 -> Word_Mux_7/7  "Stack"
  Align101/16 -> Bus Creator30/1
  Align101/15 -> Bus Creator30/2
  Align101/14 -> Bus Creator30/3
  Align101/13 -> Bus Creator30/4
  Align101/12 -> Bus Creator30/5
  Align101/11 -> Bus Creator30/6
  Align101/10 -> Bus Creator30/7
  Align101/9 -> Bus Creator30/8
  Align101/8 -> Bus Creator30/9
  Align101/7 -> Bus Creator30/10
  Align101/6 -> Bus Creator30/11
  Align101/5 -> Bus Creator30/12
  Align101/4 -> Bus Creator30/13
  Align101/3 -> Bus Creator30/14
  Align101/2 -> Bus Creator30/15
  Align101/1 -> Bus Creator30/16
  Bus Creator30/1 -> Mux_4/8  "Stack"
  Align95/8 -> Bus Creator28/1
  Align95/7 -> Bus Creator28/2
  Align95/6 -> Bus Creator28/3
  Align95/5 -> Bus Creator28/4
  Align95/4 -> Bus Creator28/5
  Align95/3 -> Bus Creator28/6
  Align95/2 -> Bus Creator28/7
  Align95/1 -> Bus Creator28/8
  Segment_Register/1(AddrOut(2B)) -> Bus Selector10/1  "Segment_Register"
  Bus Selector10/16 -> Align93/1  "<b00>"
  Bus Selector10/15 -> Align93/2  "<b01>"
  Bus Selector10/14 -> Align93/3  "<b02>"
  Bus Selector10/13 -> Align93/4  "<b03>"
  Bus Selector10/12 -> Align93/5  "<b04>"
  Bus Selector10/11 -> Align93/6  "<b05>"
  Bus Selector10/10 -> Align93/7  "<b06>"
  Bus Selector10/9 -> Align93/8  "<b07>"
  Bus Selector10/8 -> Align93/9  "<b08>"
  Bus Selector10/7 -> Align93/10  "<b09>"
  Bus Selector10/6 -> Align93/11  "<b10>"
  Bus Selector10/5 -> Align93/12  "<b11>"
  Bus Selector10/4 -> Align93/13  "<b12>"
  Bus Selector10/3 -> Align93/14  "<b13>"
  Bus Selector10/2 -> Align93/15  "<b14>"
  Bus Selector10/1 -> Align93/16  "<b15>"
  Align93/16 -> Bus Creator29/1
  Align93/15 -> Bus Creator29/2
  Align93/14 -> Bus Creator29/3
  Align93/13 -> Bus Creator29/4
  Align93/12 -> Bus Creator29/5
  Align93/11 -> Bus Creator29/6
  Align93/10 -> Bus Creator29/7
  Align93/9 -> Bus Creator29/8
  Align93/8 -> Bus Creator29/9
  Align93/7 -> Bus Creator29/10
  Align93/6 -> Bus Creator29/11
  Align93/5 -> Bus Creator29/12
  Align93/4 -> Bus Creator29/13
  Align93/3 -> Bus Creator29/14
  Align93/2 -> Bus Creator29/15
  Align93/1 -> Bus Creator29/16
  Bus Creator29/1 -> Word_Mux_4/3
